simulink model "Battery_SOC"  (R2024b)
settings: Solver=VariableStepAuto  StartTime=0.0  StopTime=descrete_time  RelTol=1e-3
values from neighbouring files (symbols this model uses):
  Cn = 2.3 *3600    (= 8280)    [battery_source_of_charge.m]
  I = 2.3    [battery_source_of_charge.m]
  OCV = Data(:,2)    [battery_source_of_charge.m]
  R_Charge = Data(:,3)    [battery_source_of_charge.m]
  R_Discharge = Data(:,4)    [battery_source_of_charge.m]
  SOC = Data(:,1)    [battery_source_of_charge.m]
settings Model: Creator=vishwanth  LastModifiedBy=vishwanth

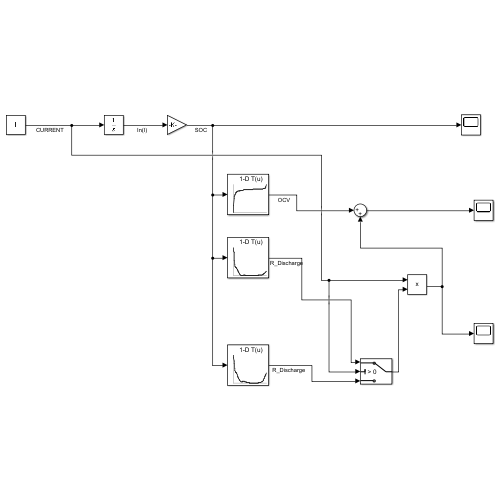
[thumbnail: Simulink's stored preview of the top-level diagram]
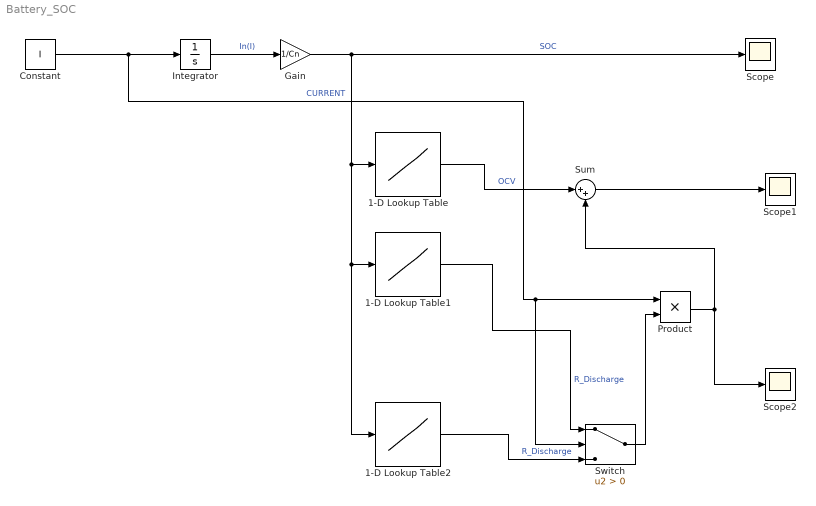
== system Battery_SOC ==
  1-D Lookup Table : Lookup_n-D  NumberOfTableDimensions=1  BreakpointsForDimension1=SOC  Table=OCV  InternalRulePriority=Speed  RndMeth=Simplest
  1-D Lookup Table1 : Lookup_n-D  NumberOfTableDimensions=1  BreakpointsForDimension1=SOC  Table=R_Discharge  InternalRulePriority=Speed  RndMeth=Simplest
  1-D Lookup Table2 : Lookup_n-D  NumberOfTableDimensions=1  BreakpointsForDimension1=SOC  Table=R_Charge  InternalRulePriority=Speed  RndMeth=Simplest
  Constant : Constant  Value=I
  Gain : Gain  Gain=1/Cn
  Integrator : Integrator
  Product : Product
  Scope : Scope
  Scope1 : Scope
  Scope2 : Scope
  Sum : Sum  Inputs=|++
  Switch : Switch  Criteria=u2 > Threshold  SaturateOnIntegerOverflow=off  InputSameDT=off
  wires:
  Constant/1 -> Switch/2, Product/1, Integrator/1  "CURRENT"
  Integrator/1 -> Gain/1  "In(I)"
  Gain/1 -> Scope/1, 1-D Lookup Table2/1, 1-D Lookup Table1/1, 1-D Lookup Table/1  "SOC"
  1-D Lookup Table1/1 -> Switch/1  "R_Discharge"
  Product/1 -> Scope2/1, Sum/2
  1-D Lookup Table/1 -> Sum/1  "OCV"
  Sum/1 -> Scope1/1
  1-D Lookup Table2/1 -> Switch/3  "R_Discharge"
  Switch/1 -> Product/2
